simulink model "Pcontrol_old"  (R2019a)
settings: Solver=VariableStepAuto  StartTime=0.0  StopTime=inf  MaxStep=1e-3  RelTol=1e-3
model workspace (MAT data in the model file):
  temp = 23
  temp_sens = 20
libraries: dspnetwork x2, simulink x1
settings Model: Creator=adria  LastModifiedBy=marcu

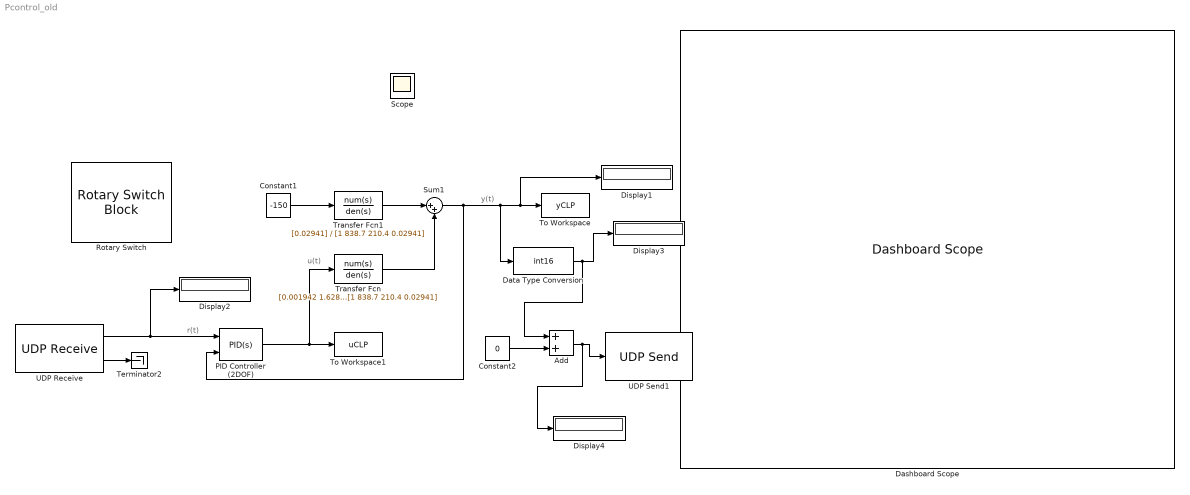
== system Pcontrol_old ==
  note: r(t)
  note: y(t)
  note: u(t)
  Add : Sum
  Constant1 : Constant  Value=-150
  Constant2 : Constant  Value=0
  Dashboard Scope : DashboardScope  Ymin=-200  Ymax=1000  WebBlockId=22
  Data Type Conversion : DataTypeConversion  OutMin=0  OutDataTypeStr=int16  ConvertRealWorld=Stored Integer (SI)  RndMeth=Nearest  SaturateOnIntegerOverflow=on  LockScale=on
  Display{1..4} (4 alike) : Display
  PID Controller (2DOF) : simulink/Continuous/PID Controller (2DOF)  Controller=PID  Form=Parallel  TimeDomain=Continuous-time  SampleTime=-1  IntegratorMethod=Forward Euler  FilterMethod=Forward Euler  ControllerParametersSource=internal  P=4  I=0.01  D=0  UseFilter=on  N=100  b=1  c=1  TunerSelectOption=Transfer Function Based (PID Tuner App)  InitialConditionSource=internal  InitialConditionForIntegrator=0  InitialConditionForFilter=0  DifferentiatorICPrevScaledInput=0  ExternalReset=none  TrackingMode=off  Kt=1  LimitOutput=off  UpperSaturationLimit=inf  LowerSaturationLimit=-inf  LinearizeAsGain=on  AntiWindupMode=none  Kb=1  POutMin=[]  POutMax=[]  IOutMin=[]  IOutMax=[]  DOutMin=[]  DOutMax=[]  NOutMin=[]  NOutMax=[]  bOutMin=[]  bOutMax=[]  cOutMin=[]  cOutMax=[]  SumOutMin=[]  SumOutMax=[]  SaturationOutMin=[]  SaturationOutMax=[]  PParamMin=[]  PParamMax=[]  IParamMin=[]  IParamMax=[]  DParamMin=[]  DParamMax=[]  NParamMin=[]  NParamMax=[]  bParamMin=[]  bParamMax=[]  cParamMin=[]  cParamMax=[]  KbParamMin=[]  KbParamMax=[]  KtParamMin=[]  KtParamMax=[]  KbOutMin=[]  KbOutMax=[]  KtOutMin=[]  KtOutMax=[]  IntegratorOutMin=[]  IntegratorOutMax=[]  FilterOutMin=[]  FilterOutMax=[]  SumI1OutMin=[]  SumI1OutMax=[]  SumI2OutMin=[]  SumI2OutMax=[]  SumI3OutMin=[]  SumI3OutMax=[]  SumI4OutMin=[]  SumI4OutMax=[]  SumDOutMin=[]  SumDOutMax=[]  Sum1OutMin=[]  Sum1OutMax=[]  Sum2OutMin=[]  Sum2OutMax=[]  Sum3OutMin=[]  Sum3OutMax=[]  DifferentiatorOutMin=[]  DifferentiatorOutMax=[]  FilterDiffOutCoefMin=[]  FilterDiffOutCoefMax=[]  ReciprocalOutMin=[]  ReciprocalOutMax=[]  SumDenOutMin=[]  SumDenOutMax=[]  SumNumOutMin=[]  SumNumOutMax=[]  DivideOutMin=[]  DivideOutMax=[]  IntegratorContinuousStateAttributes=''  IntegratorStateMustResolveToSignalObject=off  IntegratorRTWStateStorageClass=Auto  FilterContinuousStateAttributes=''  FilterStateMustResolveToSignalObject=off  FilterRTWStateStorageClass=Auto  ParallelPVariant=InternalParameters  IdealPVariant=Disabled  IVariant=InternalParameters  DVariant=InternalParameters  bVariant=InternalParameters  cVariant=InternalParameters  IntegratorVariant=Continuous  SatVariant=Disabled  AWVariant=Passthrough  PCopyVariant=Disabled  TRVariant=Disabled  FdbkBlocksVariant=Forward  IdealPFdbkVariant=Disabled  SatFdbkVariant=Disabled  DerivativeFilterVariant=ContFilter  NVariant=InternalParameters  NCopyVariant=Disabled  FilterICVariant=InternalICsFilter  IntegratorICVariant=InternalICs  ExternalResetVariant=Disabled  TRSumVariant=Passthrough  SumFdbkVariant=Disabled  SumVariant=Sum_PID
  Rotary Switch : RotarySwitchBlock  WebBlockId=27
      settings: Values={{'-150', '-130', '-100', '-70', '-20', '0', '10', '20'}, [-150 -130 -100 -70 -20 0 10 20]}
  Sum1 : Sum  Inputs=|++
  Terminator2 : Terminator
  To Workspace : ToWorkspace  VariableName=yCLP  SaveFormat=Structure With Time  SampleTime=-1
  To Workspace1 : ToWorkspace  VariableName=uCLP  SaveFormat=Structure With Time  SampleTime=-1
  Transfer Fcn : TransferFcn  Numerator=[0.001942 1.628 0.4083]  Denominator=[1 838.7 210.4 0.02941]
  Transfer Fcn1 : TransferFcn  Numerator=[0.02941]  Denominator=[1 838.7 210.4 0.02941]
  UDP Receive : dspnetwork/UDP Receive  localURL='0.0.0.0'  localPort=10002  remoteURL='0.0.0.0'  remotePort=-1  recvBufferSize=2  dims=1  signalDatatype=int16  isComplex=off  isVarSize=off  showBlockingTime=off  blockingTime=0  sampletime=0.1  blockPlatform=LINUX
      settings: SourceProductName=Simulink
  UDP Send1 : dspnetwork/UDP Send  remoteURL='localhost'  remotePort=10001  localURL='255.255.255.255'  localPortSource=Automatically determine  localPort=-1  sampletime=-1  blockPlatform=LINUX  separateLengthPort=0
      settings: SourceProductName=Simulink
  Scope : Scope
  wires:
  Transfer Fcn/1 -> Sum1/2
  Constant1/1 -> Transfer Fcn1/1
  Transfer Fcn1/1 -> Sum1/1
  PID Controller (2DOF)/1 -> Transfer Fcn/1, To Workspace1/1
  Sum1/1 -> PID Controller (2DOF)/2, Data Type Conversion/1, Display1/1, To Workspace/1
  UDP Receive/2 -> Terminator2/1
  Data Type Conversion/1 -> Add/1, Display3/1
  Constant2/1 -> Add/2
  Add/1 -> Display4/1, UDP Send1/1
  UDP Receive/1 -> PID Controller (2DOF)/1, Display2/1
